simulink subsystem "stewart_strut"  (R2025b)
settings: Solver=VariableStepAuto  StartTime=0.0  StopTime=10.0  RelTol=1e-3
undefined symbols (not defined in the file): DiscIntNeverNeededParam, i, lengthServoConfig, stewart, X, Y, Z
libraries: sm_lib x53, nesl_utility x39
(part 1 of 3)
settings Model: Creator=thomas  LastModifiedBy=David_X
settings SolverCC: AlgebraicLoopSolver=TrustRegion
settings DebuggingCC: UnconnectedInputMsg=warning  UnconnectedOutputMsg=warning  UnconnectedLineMsg=warning
settings ModelReferenceCC: EnableRefExpFcnMdlSchedulingChecks=on
settings RTWCC: GPUComputeCapability=3.5

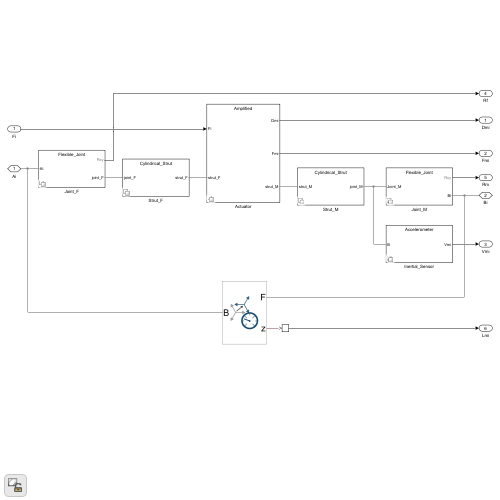
[thumbnail: Simulink's stored preview of the top-level diagram]
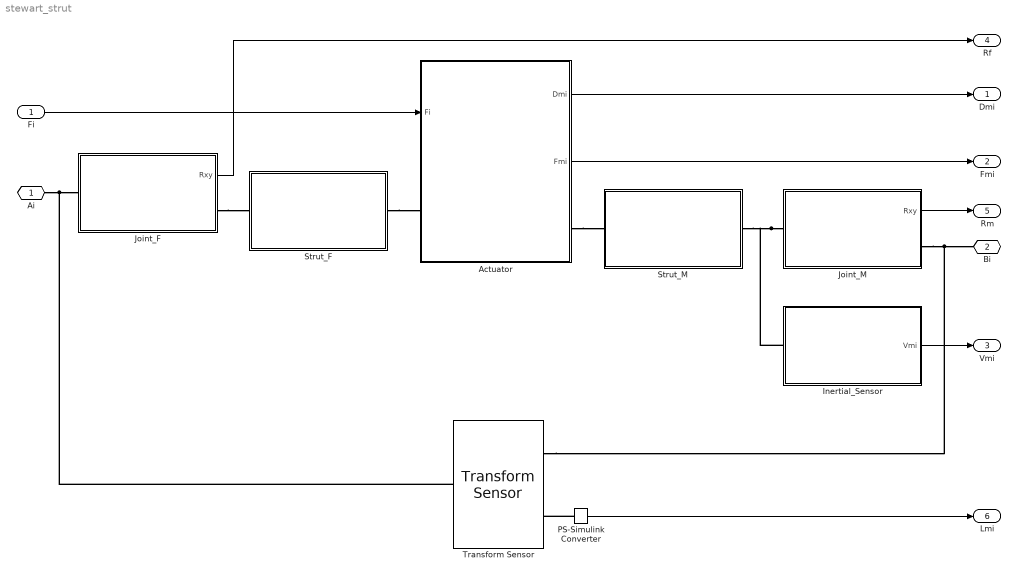
== system stewart_strut ==
  Fi : Inport  Unit=N
  Actuator : Subsystem  Variant=on  VariantControl=Variant1
  Inertial_Sensor : Subsystem  Variant=on  VariantControl=Variant1
  Joint_F : Subsystem  Variant=on  VariantControl=Variant1
  Joint_M : Subsystem  Variant=on  VariantControl=Variant1
  PS-Simulink Converter : nesl_utility/PS-Simulink Converter  PhysicalDomain=network_engine_domain  SubClassName=ps_output  LeftPortType=input  RightPortType=output  PseudoPeriodic=off  Frequencies=[]  VectorFormat=1-D array  Unit=inherit  AffineConversion=off
  Strut_F : Subsystem  Variant=on  VariantControl=Variant1
  Strut_M : Subsystem  Variant=on  VariantControl=Variant1
  Transform Sensor : sm_lib/Frames and Transforms/Transform Sensor  MeasurementFrame=Base  RotationSequence=XYX  SenseAngle=off  SenseAxis=off  SenseQ=off  SenseR=off  SenseRotationSequence=off  SenseOmegaX=off  SenseOmegaY=off  SenseOmegaZ=off  SenseOmega=off  SenseQDot=off  SenseRDot=off  SenseRotationSequenceDot=off  SenseAlphaX=off  SenseAlphaY=off  SenseAlphaZ=off  SenseAlpha=off  SenseQDDot=off  SenseRDDot=off  SenseX=off  SenseY=off  SenseZ=on  SenseXYZ=off  SenseRad=off  SenseAzim=off  SenseDist=off  SenseInc=off  SenseXDot=off  SenseYDot=off  SenseZDot=off  SenseXYZDot=off  SenseRadDot=off  SenseAzimDot=off  SenseDistDot=off  SenseIncDot=off  SenseXDDot=off  SenseYDDot=off  SenseZDDot=off  SenseXYZDDot=off  SenseRadDDot=off  SenseAzimDDot=off  SenseDistDDot=off  SenseIncDDot=off
  Ai : PMIOPort  Side=Left
  Bi : PMIOPort  Port=2  Side=Right
  Dmi : Outport
  Fmi : Outport  Port=2
  Vmi : Outport  Port=3
  Rf : Outport  Port=4
  Rm : Outport  Port=5
  Lmi : Outport  Port=6
  wires:
  Inertial_Sensor/1(Vmi) -> Vmi/1
  Actuator/1(Dmi) -> Dmi/1
  Fi/1 -> Actuator/1(Fi)
  Actuator/2(Fmi) -> Fmi/1
  Joint_M/1(Rxy) -> Rm/1
  Joint_F/1(Rxy) -> Rf/1
  PS-Simulink Converter/1 -> Lmi/1
  connections:
  Transform Sensor/LConn1 -- Ai/RConn1 -- Joint_F/LConn1
  Transform Sensor/RConn1 -- Joint_M/RConn1 -- Bi/RConn1
  Joint_M/LConn1 -- Strut_M/RConn1 -- Inertial_Sensor/LConn1
  Actuator/RConn1 -- Strut_M/LConn1
  Joint_F/RConn1 -- Strut_F/LConn1
  Strut_F/RConn1 -- Actuator/LConn1
  PS-Simulink Converter/LConn1 -- Transform Sensor/RConn2

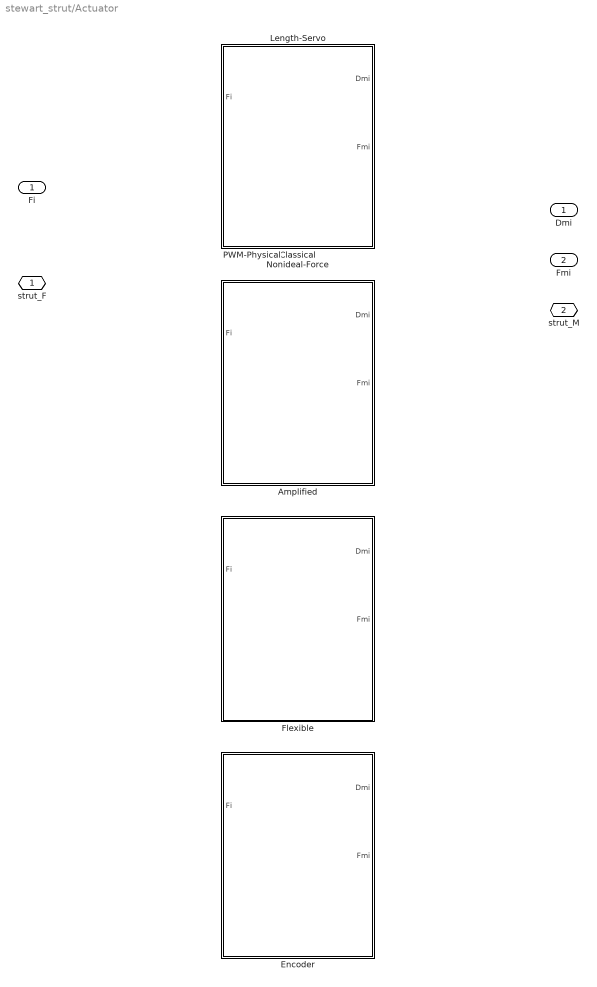
== system stewart_strut/Actuator ==
  Fi : Inport
  Amplified : Subsystem  VariantControl=stewart.actuators.type==2
  Classical : Subsystem  VariantControl=stewart.actuators.type==1
  Encoder : Subsystem  VariantControl=stewart.actuators.type==4
  Flexible : Subsystem  VariantControl=stewart.actuators.type==3
  Length-Servo : Subsystem  VariantControl=stewart.actuators.type==5
  Nonideal-Force : Subsystem  VariantControl=stewart.actuators.type==7
  PWM-Physical : Subsystem  VariantControl=stewart.actuators.type==6
  strut_F : PMIOPort  Side=Left
  strut_M : PMIOPort  Port=2  Side=Right
  Dmi : Outport
  Fmi : Outport  Port=2

== system stewart_strut/Inertial_Sensor ==
  Accelerometer : Subsystem  VariantControl=stewart.sensors.inertial.type == 2
  Geophone : Subsystem  VariantControl=stewart.sensors.inertial.type == 1
  None : Subsystem  VariantControl=stewart.sensors.inertial.type == 3
  B : PMIOPort  Side=Left
  Vmi : Outport

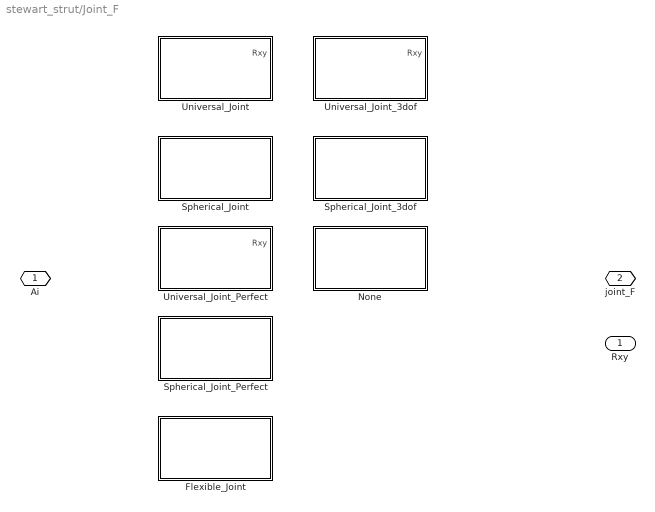
== system stewart_strut/Joint_F ==
  Flexible_Joint : Subsystem  VariantControl=stewart.joints_F.type == 5
  None : Subsystem  VariantControl=stewart.joints_F.type == 10
  Spherical_Joint : Subsystem  VariantControl=stewart.joints_F.type == 2
  Spherical_Joint_3dof : Subsystem  VariantControl=stewart.joints_F.type == 7
  Spherical_Joint_Perfect : Subsystem  VariantControl=stewart.joints_F.type == 4
  Universal_Joint : Subsystem  VariantControl=stewart.joints_F.type == 1
  Universal_Joint_3dof : Subsystem  VariantControl=stewart.joints_F.type == 6
  Universal_Joint_Perfect : Subsystem  VariantControl=stewart.joints_F.type == 3
  Ai : PMIOPort  Side=Left
  joint_F : PMIOPort  Port=2  Side=Right
  Rxy : Outport

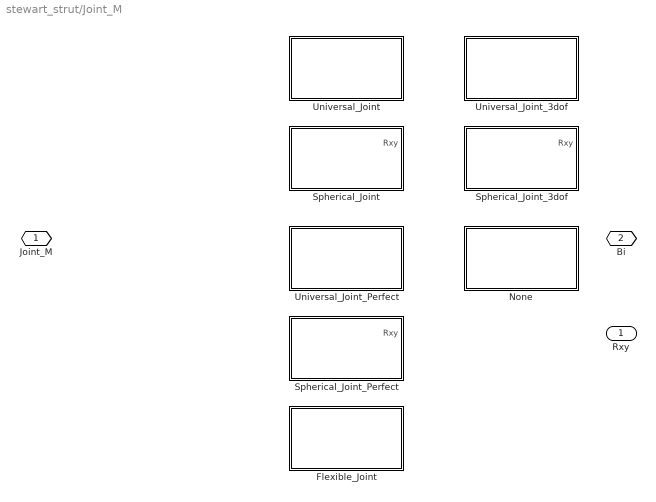
== system stewart_strut/Joint_M ==
  Flexible_Joint : Subsystem  VariantControl=stewart.joints_M.type == 5
  None : Subsystem  VariantControl=stewart.joints_M.type == 10
  Spherical_Joint : Subsystem  VariantControl=stewart.joints_M.type == 2
  Spherical_Joint_3dof : Subsystem  VariantControl=stewart.joints_M.type == 7
  Spherical_Joint_Perfect : Subsystem  VariantControl=stewart.joints_M.type == 4
  Universal_Joint : Subsystem  VariantControl=stewart.joints_M.type == 1
  Universal_Joint_3dof : Subsystem  VariantControl=stewart.joints_M.type == 6
  Universal_Joint_Perfect : Subsystem  VariantControl=stewart.joints_M.type == 3
  Joint_M : PMIOPort  Side=Left
  Bi : PMIOPort  Port=2  Side=Right
  Rxy : Outport

== system stewart_strut/Strut_F ==
  Cylindrical_Strut : Subsystem  VariantControl=stewart.struts_F.type == 1
  None : Subsystem  VariantControl=stewart.struts_F.type == 2
  Null : Subsystem  VariantControl=stewart.struts_F.type == 3
  joint_F : PMIOPort  Side=Left
  strut_F : PMIOPort  Port=2  Side=Right

== system stewart_strut/Strut_M ==
  Cylindrical_Strut : Subsystem  VariantControl=stewart.struts_F.type == 1
  None : Subsystem  VariantControl=stewart.struts_F.type == 2
  Null : Subsystem  VariantControl=stewart.struts_F.type == 3
  strut_M : PMIOPort  Side=Left
  joint_M : PMIOPort  Port=2  Side=Right

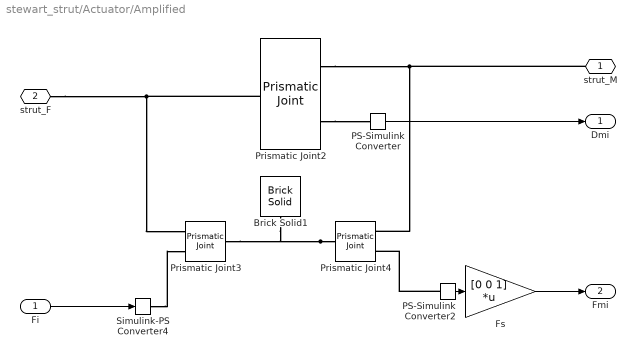
== system stewart_strut/Actuator/Amplified ==
  Fi : Inport
  Brick Solid1 : sm_lib/Body Elements/Brick Solid  BrickDimensions=[1 1 1.5]  BrickDimensionsUnits=cm  ExportEntireGeometry=off  InertiaType=CalculateFromGeometry  BasedOnType=Mass  Density=1000  DensityUnits=kg/m^3  Mass=0.001  MassUnits=kg  CenterOfMass=[0 0 0]  CenterOfMassUnits=m  MomentsOfInertia=[1 1 1]  MomentsOfInertiaUnits=kg*m^2  ProductsOfInertia=[0 0 0]  ProductsOfInertiaUnits=kg*m^2  GraphicType=FromGeometry  MarkerShape=Sphere  MarkerSize=10  GraphicVisPropType=SimpleVisualProperties  GraphicDiffuseColor=[0.5 0.5 0.5]  GraphicOpacity=1.0  GraphicSpecularColor=[0.5 0.5 0.5 1.0]  GraphicAmbientColor=[0.15 0.15 0.15 1.0]  GraphicEmissiveColor=[0.0 0.0 0.0 1.0]  GraphicShininess=75  DoExposeReferenceFrame=on  SerializedFrames=<Frames/>
  Fs : Gain  Gain=[0 0 1]  Multiplication=Matrix(K*u)
  PS-Simulink Converter : nesl_utility/PS-Simulink Converter  PhysicalDomain=network_engine_domain  SubClassName=ps_output  LeftPortType=input  RightPortType=output  PseudoPeriodic=off  Frequencies=[]  VectorFormat=1-D array  Unit=m  AffineConversion=off
  PS-Simulink Converter2 : nesl_utility/PS-Simulink Converter  PhysicalDomain=network_engine_domain  SubClassName=ps_output  LeftPortType=input  RightPortType=output  PseudoPeriodic=off  Frequencies=[]  VectorFormat=1-D array  Unit=N  AffineConversion=off
  Prismatic Joint2 : sm_lib/Joints/Prismatic Joint  JointMode=Normal  CompositeWrenchDir=FollowerOnBase  CompositeWrenchFrame=BaseFrame  SenseConstraintForce=off  SenseConstraintTorque=off  SenseTotalForce=off  SenseTotalTorque=off  PositionTargetSpecify=off  PositionTargetPriority=High  PositionTargetValue=0  PositionTargetValueUnits=m  VelocityTargetSpecify=off  VelocityTargetPriority=High  VelocityTargetValue=0  VelocityTargetValueUnits=m/s  EquilibriumPosition=stewart.actuators.Leq(i)  EquilibriumPositionUnits=m  SpringStiffness=stewart.actuators.K1(i)  SpringStiffnessUnits=N/m  DampingCoefficient=stewart.actuators.C1(i)  DampingCoefficientUnits=N/(m/s)  LowerLimitSpecify=off  LowerLimitBound=-1  LowerLimitBoundUnits=m  LowerLimitStiffness=1e6  LowerLimitStiffnessUnits=N/m  LowerLimitDamping=1e3  LowerLimitDampingUnits=N/(m/s)  LowerLimitTransitionRegionWidth=1e-4  LowerLimitTransitionRegionWidthUnits=m  UpperLimitSpecify=off  UpperLimitBound=1  UpperLimitBoundUnits=m  UpperLimitStiffness=1e6  UpperLimitStiffnessUnits=N/m  UpperLimitDamping=1e3  UpperLimitDampingUnits=N/(m/s)  UpperLimitTransitionRegionWidth=1e-4  UpperLimitTransitionRegionWidthUnits=m  TorqueActuationMode=NoTorque  MotionActuationMode=ComputedMotion  SensePosition=on  SenseVelocity=off  SenseAcceleration=off  SenseTorqueForce=off  SenseLowerLimitTorqueForce=off  SenseUpperLimitTorqueForce=off
  Prismatic Joint3 : sm_lib/Joints/Prismatic Joint  JointMode=Normal  CompositeWrenchDir=FollowerOnBase  CompositeWrenchFrame=BaseFrame  SenseConstraintForce=off  SenseConstraintTorque=off  SenseTotalForce=off  SenseTotalTorque=off  PositionTargetSpecify=off  PositionTargetPriority=Low  PositionTargetValue=0  PositionTargetValueUnits=m  VelocityTargetSpecify=off  VelocityTargetPriority=High  VelocityTargetValue=0  VelocityTargetValueUnits=m/s  EquilibriumPosition=0  EquilibriumPositionUnits=m  SpringStiffness=stewart.actuators.Ka(i)  SpringStiffnessUnits=N/m  DampingCoefficient=0  DampingCoefficientUnits=N/(m/s)  LowerLimitSpecify=off  LowerLimitBound=-1  LowerLimitBoundUnits=m  LowerLimitStiffness=1e6  LowerLimitStiffnessUnits=N/m  LowerLimitDamping=1e3  LowerLimitDampingUnits=N/(m/s)  LowerLimitTransitionRegionWidth=1e-4  LowerLimitTransitionRegionWidthUnits=m  UpperLimitSpecify=off  UpperLimitBound=1  UpperLimitBoundUnits=m  UpperLimitStiffness=1e6  UpperLimitStiffnessUnits=N/m  UpperLimitDamping=1e3  UpperLimitDampingUnits=N/(m/s)  UpperLimitTransitionRegionWidth=1e-4  UpperLimitTransitionRegionWidthUnits=m  TorqueActuationMode=InputTorque  MotionActuationMode=ComputedMotion  SensePosition=off  SenseVelocity=off  SenseAcceleration=off  SenseTorqueForce=off  SenseLowerLimitTorqueForce=off  SenseUpperLimitTorqueForce=off
  Prismatic Joint4 : sm_lib/Joints/Prismatic Joint  JointMode=Normal  CompositeWrenchDir=FollowerOnBase  CompositeWrenchFrame=BaseFrame  SenseConstraintForce=off  SenseConstraintTorque=off  SenseTotalForce=on  SenseTotalTorque=off  PositionTargetSpecify=off  PositionTargetPriority=Low  PositionTargetValue=0  PositionTargetValueUnits=m  VelocityTargetSpecify=off  VelocityTargetPriority=High  VelocityTargetValue=0  VelocityTargetValueUnits=m/s  EquilibriumPosition=0  EquilibriumPositionUnits=m  SpringStiffness=stewart.actuators.Ke(i)  SpringStiffnessUnits=N/m  DampingCoefficient=0  DampingCoefficientUnits=N/(m/s)  LowerLimitSpecify=off  LowerLimitBound=-1  LowerLimitBoundUnits=m  LowerLimitStiffness=1e6  LowerLimitStiffnessUnits=N/m  LowerLimitDamping=1e3  LowerLimitDampingUnits=N/(m/s)  LowerLimitTransitionRegionWidth=1e-4  LowerLimitTransitionRegionWidthUnits=m  UpperLimitSpecify=off  UpperLimitBound=1  UpperLimitBoundUnits=m  UpperLimitStiffness=1e6  UpperLimitStiffnessUnits=N/m  UpperLimitDamping=1e3  UpperLimitDampingUnits=N/(m/s)  UpperLimitTransitionRegionWidth=1e-4  UpperLimitTransitionRegionWidthUnits=m  TorqueActuationMode=NoTorque  MotionActuationMode=ComputedMotion  SensePosition=off  SenseVelocity=off  SenseAcceleration=off  SenseTorqueForce=off  SenseLowerLimitTorqueForce=off  SenseUpperLimitTorqueForce=off
  Simulink-PS Converter4 : nesl_utility/Simulink-PS Converter  PhysicalDomain=network_engine_domain  SubClassName=ps_input  LeftPortType=input  RightPortType=output  PseudoPeriodic=off  Frequencies=[]  NoiseDistribution=none  NoiseParameters=[]  Unit=N  AffineConversion=off  FilteringAndDerivatives=provide  SimscapeFilterOrder=1  InputFilterTimeConstant=0.001  UdotUserProvided=0
  strut_M : PMIOPort  Side=Right
  strut_F : PMIOPort  Port=2  Side=Left
  Dmi : Outport
  Fmi : Outport  Port=2
  wires:
  PS-Simulink Converter/1 -> Dmi/1
  PS-Simulink Converter2/1 -> Fs/1
  Fi/1 -> Simulink-PS Converter4/1
  Fs/1 -> Fmi/1
  connections:
  strut_M/RConn1 -- Prismatic Joint2/RConn1 -- Prismatic Joint4/RConn1
  Prismatic Joint2/LConn1 -- Prismatic Joint3/LConn1 -- strut_F/RConn1
  PS-Simulink Converter2/LConn1 -- Prismatic Joint4/RConn2
  Simulink-PS Converter4/RConn1 -- Prismatic Joint3/LConn2
  Prismatic Joint2/RConn2 -- PS-Simulink Converter/LConn1
  Prismatic Joint4/LConn1 -- Prismatic Joint3/RConn1 -- Brick Solid1/RConn1

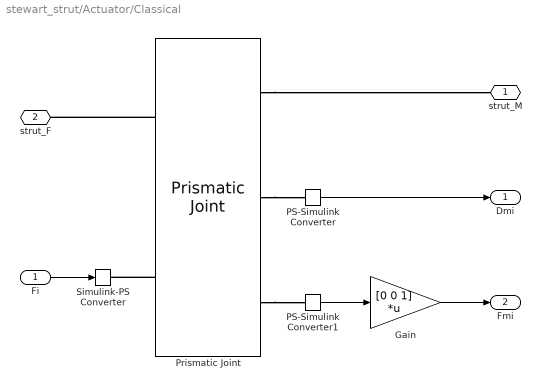
== system stewart_strut/Actuator/Classical ==
  Fi : Inport
  Gain : Gain  Gain=[0 0 1]  Multiplication=Matrix(K*u)
  PS-Simulink Converter : nesl_utility/PS-Simulink Converter  PhysicalDomain=network_engine_domain  SubClassName=ps_output  LeftPortType=input  RightPortType=output  PseudoPeriodic=off  Frequencies=[]  VectorFormat=1-D array  Unit=m  AffineConversion=off
  PS-Simulink Converter1 : nesl_utility/PS-Simulink Converter  PhysicalDomain=network_engine_domain  SubClassName=ps_output  LeftPortType=input  RightPortType=output  PseudoPeriodic=off  Frequencies=[]  VectorFormat=1-D array  Unit=N  AffineConversion=on
  Prismatic Joint : sm_lib/Joints/Prismatic Joint  JointMode=Normal  CompositeWrenchDir=BaseOnFollower  CompositeWrenchFrame=BaseFrame  SenseConstraintForce=off  SenseConstraintTorque=off  SenseTotalForce=on  SenseTotalTorque=off  PositionTargetSpecify=on  PositionTargetPriority=High  PositionTargetValue=stewart.actuators.Leq(i)  PositionTargetValueUnits=m  VelocityTargetSpecify=off  VelocityTargetPriority=High  VelocityTargetValue=0  VelocityTargetValueUnits=m/s  EquilibriumPosition=stewart.actuators.Leq(i)  EquilibriumPositionUnits=m  SpringStiffness=stewart.actuators.K(i)  SpringStiffnessUnits=N/m  DampingCoefficient=stewart.actuators.C(i)  DampingCoefficientUnits=N/(m/s)  LowerLimitSpecify=off  LowerLimitBound=-1  LowerLimitBoundUnits=m  LowerLimitStiffness=1e6  LowerLimitStiffnessUnits=N/m  LowerLimitDamping=1e3  LowerLimitDampingUnits=N/(m/s)  LowerLimitTransitionRegionWidth=1e-4  LowerLimitTransitionRegionWidthUnits=m  UpperLimitSpecify=off  UpperLimitBound=1  UpperLimitBoundUnits=m  UpperLimitStiffness=1e6  UpperLimitStiffnessUnits=N/m  UpperLimitDamping=1e3  UpperLimitDampingUnits=N/(m/s)  UpperLimitTransitionRegionWidth=1e-4  UpperLimitTransitionRegionWidthUnits=m  TorqueActuationMode=InputTorque  MotionActuationMode=ComputedMotion  SensePosition=on  SenseVelocity=off  SenseAcceleration=off  SenseTorqueForce=off  SenseLowerLimitTorqueForce=off  SenseUpperLimitTorqueForce=off
  Simulink-PS Converter : nesl_utility/Simulink-PS Converter  PhysicalDomain=network_engine_domain  SubClassName=ps_input  LeftPortType=input  RightPortType=output  PseudoPeriodic=off  Frequencies=[]  NoiseDistribution=none  NoiseParameters=[]  Unit=N  AffineConversion=off  FilteringAndDerivatives=provide  SimscapeFilterOrder=1  InputFilterTimeConstant=0.001  UdotUserProvided=0
  strut_M : PMIOPort  Side=Right
  strut_F : PMIOPort  Port=2  Side=Left
  Dmi : Outport
  Fmi : Outport  Port=2
  wires:
  Gain/1 -> Fmi/1
  Fi/1 -> Simulink-PS Converter/1
  PS-Simulink Converter1/1 -> Gain/1
  PS-Simulink Converter/1 -> Dmi/1
  connections:
  Prismatic Joint/RConn3 -- PS-Simulink Converter1/LConn1
  Prismatic Joint/RConn2 -- PS-Simulink Converter/LConn1
  Prismatic Joint/RConn1 -- strut_M/RConn1
  Prismatic Joint/LConn2 -- Simulink-PS Converter/RConn1
  Prismatic Joint/LConn1 -- strut_F/RConn1

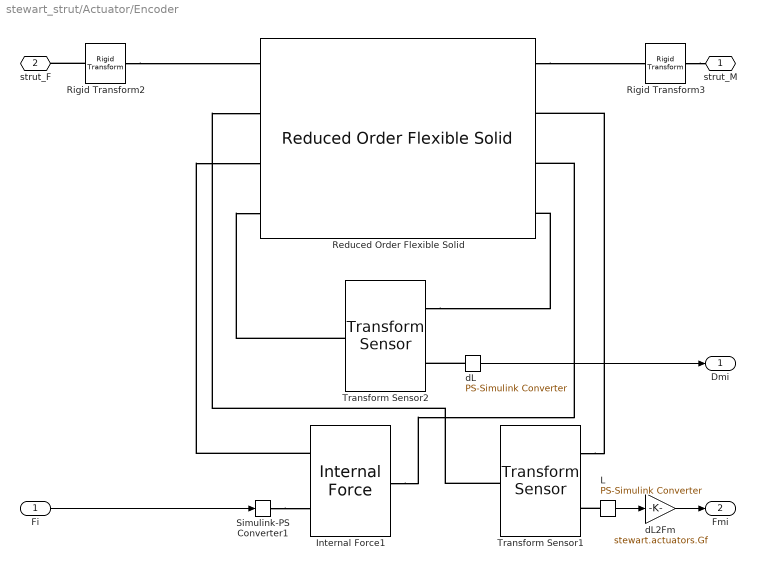
== system stewart_strut/Actuator/Encoder ==
  Fi : Inport
  Internal Force1 : sm_lib/Forces and Torques/Internal Force
  L : nesl_utility/PS-Simulink Converter  PhysicalDomain=network_engine_domain  SubClassName=ps_output  LeftPortType=input  RightPortType=output  PseudoPeriodic=off  Frequencies=[]  VectorFormat=1-D array  Unit=m  AffineConversion=off
  Reduced Order Flexible Solid : sm_lib/Body Elements/Flexible Bodies/Reduced Order Flexible Solid  UnitSystemType=SI  LengthUnit=m  MassUnit=kg  TimeUnit=s  NumberOfInterfaceFrames=8  InterfaceFrameOrigins=stewart.actuators.n_xyz  InterfaceFrameOrientations=repmat([1 0 0 0],8,1)  StiffnessMatrix=stewart.actuators.Km  MassMatrix=stewart.actuators.Mm  DampingType=UniformModal  ProportionalDampingAlpha=1e-6  ProportionalDampingBeta=3e-6  UniformModalDampingRatio=stewart.actuators.xi  DampingMatrix=[]  ReferenceConditionsType=LinearizedMeanAxes  DoExposeReferenceFrame=off  ReductionType=None  NumRetainedModes=1  GraphicType=PartitionedGeometry  GeomFileName=./mat/strut_encoder.step  GeomUnitType=FromFile  VisRecursionLimit=3  GraphicVertexCoordinates=[]  GraphicFacetVertexIndices=[]  GraphicReconstructionMatrix=[]  GraphicVisPropType=SimpleVisualProperties  GraphicDiffuseColor=[0.2 0.4 1.0]  GraphicOpacity=1.0  GraphicSpecularColor=[0.5 0.5 0.5 1.0]  GraphicAmbientColor=[0.15 0.15 0.15 1.0]  GraphicEmissiveColor=[0.0 0.0 0.0 1.0]  GraphicShininess=75
  Rigid Transform2 : sm_lib/Frames and Transforms/Rigid Transform  RotationMethod=None  FollAlignAxisA=+X  BaseAlignAxisA=+Y  FollAlignAxisB=+Y  BaseAlignAxisB=+Z  RotationStandardAxis=+Z  RotationAngle=0.0  RotationAngleUnits=deg  RotationArbitraryAxis=[0 0 1]  RotationSequenceAxes=FollowerAxes  RotationSequence=XYX  RotationSequenceAngles=[0 0 0]  RotationSequenceAnglesUnits=deg  RotationMatrix=[1 0 0; 0 1 0; 0 0 1]  Quaternion=[1 0 0 0]  TranslationMethod=StandardAxis  TranslationCartesianOffset=[0 0 0]  TranslationCartesianOffsetUnits=m  TranslationStandardAxis=+Z  TranslationStandardOffset=stewart.actuators.ax_off  TranslationStandardOffsetUnits=m  TranslationROffset=0  TranslationROffsetUnits=m  TranslationThetaOffset=0  TranslationThetaOffsetUnits=deg  TranslationZOffset=0  TranslationZOffsetUnits=m
  Rigid Transform3 : sm_lib/Frames and Transforms/Rigid Transform  RotationMethod=None  FollAlignAxisA=+X  BaseAlignAxisA=+Y  FollAlignAxisB=+Y  BaseAlignAxisB=+Z  RotationStandardAxis=+Z  RotationAngle=0.0  RotationAngleUnits=deg  RotationArbitraryAxis=[0 0 1]  RotationSequenceAxes=FollowerAxes  RotationSequence=XYX  RotationSequenceAngles=[0 0 0]  RotationSequenceAnglesUnits=deg  RotationMatrix=[1 0 0; 0 1 0; 0 0 1]  Quaternion=[1 0 0 0]  TranslationMethod=StandardAxis  TranslationCartesianOffset=[0 0 0]  TranslationCartesianOffsetUnits=m  TranslationStandardAxis=+Z  TranslationStandardOffset=stewart.actuators.ax_off  TranslationStandardOffsetUnits=m  TranslationROffset=0  TranslationROffsetUnits=m  TranslationThetaOffset=0  TranslationThetaOffsetUnits=deg  TranslationZOffset=0  TranslationZOffsetUnits=m
  Simulink-PS Converter1 : nesl_utility/Simulink-PS Converter  PhysicalDomain=network_engine_domain  SubClassName=ps_input  LeftPortType=input  RightPortType=output  PseudoPeriodic=off  Frequencies=[]  NoiseDistribution=none  NoiseParameters=[]  Unit=N  AffineConversion=off  FilteringAndDerivatives=provide  SimscapeFilterOrder=1  InputFilterTimeConstant=0.001  UdotUserProvided=0
  Transform Sensor1 : sm_lib/Frames and Transforms/Transform Sensor  MeasurementFrame=Base  RotationSequence=XYX  SenseAngle=off  SenseAxis=off  SenseQ=off  SenseR=off  SenseRotationSequence=off  SenseOmegaX=off  SenseOmegaY=off  SenseOmegaZ=off  SenseOmega=off  SenseQDot=off  SenseRDot=off  SenseRotationSequenceDot=off  SenseAlphaX=off  SenseAlphaY=off  SenseAlphaZ=off  SenseAlpha=off  SenseQDDot=off  SenseRDDot=off  SenseX=on  SenseY=off  SenseZ=off  SenseXYZ=off  SenseRad=off  SenseAzim=off  SenseDist=off  SenseInc=off  SenseXDot=off  SenseYDot=off  SenseZDot=off  SenseXYZDot=off  SenseRadDot=off  SenseAzimDot=off  SenseDistDot=off  SenseIncDot=off  SenseXDDot=off  SenseYDDot=off  SenseZDDot=off  SenseXYZDDot=off  SenseRadDDot=off  SenseAzimDDot=off  SenseDistDDot=off  SenseIncDDot=off
  Transform Sensor2 : sm_lib/Frames and Transforms/Transform Sensor  MeasurementFrame=Base  RotationSequence=XYX  SenseAngle=off  SenseAxis=off  SenseQ=off  SenseR=off  SenseRotationSequence=off  SenseOmegaX=off  SenseOmegaY=off  SenseOmegaZ=off  SenseOmega=off  SenseQDot=off  SenseRDot=off  SenseRotationSequenceDot=off  SenseAlphaX=off  SenseAlphaY=off  SenseAlphaZ=off  SenseAlpha=off  SenseQDDot=off  SenseRDDot=off  SenseX=off  SenseY=off  SenseZ=on  SenseXYZ=off  SenseRad=off  SenseAzim=off  SenseDist=off  SenseInc=off  SenseXDot=off  SenseYDot=off  SenseZDot=off  SenseXYZDot=off  SenseRadDot=off  SenseAzimDot=off  SenseDistDot=off  SenseIncDot=off  SenseXDDot=off  SenseYDDot=off  SenseZDDot=off  SenseXYZDDot=off  SenseRadDDot=off  SenseAzimDDot=off  SenseDistDDot=off  SenseIncDDot=off
  dL : nesl_utility/PS-Simulink Converter  PhysicalDomain=network_engine_domain  SubClassName=ps_output  LeftPortType=input  RightPortType=output  PseudoPeriodic=off  Frequencies=[]  VectorFormat=1-D array  Unit=m  AffineConversion=off
  dL2Fm : Gain  Gain=stewart.actuators.Gf
  strut_M : PMIOPort  Side=Right
  strut_F : PMIOPort  Port=2  Side=Left
  Dmi : Outport
  Fmi : Outport  Port=2
  wires:
  dL/1 -> Dmi/1
  dL2Fm/1 -> Fmi/1
  Fi/1 -> Simulink-PS Converter1/1
  L/1 -> dL2Fm/1
  connections:
  Transform Sensor2/LConn1 -- Reduced Order Flexible Solid/RConn4
  Reduced Order Flexible Solid/LConn1 -- Rigid Transform3/LConn1
  Rigid Transform2/RConn1 -- Reduced Order Flexible Solid/RConn1
  dL/LConn1 -- Transform Sensor2/RConn2
  Transform Sensor2/RConn1 -- Reduced Order Flexible Solid/LConn4
  Transform Sensor1/RConn1 -- Reduced Order Flexible Solid/LConn2
  Transform Sensor1/LConn1 -- Reduced Order Flexible Solid/RConn2
  Internal Force1/RConn1 -- Reduced Order Flexible Solid/LConn3
  Internal Force1/LConn1 -- Reduced Order Flexible Solid/RConn3
  Rigid Transform2/LConn1 -- strut_F/RConn1
  Rigid Transform3/RConn1 -- strut_M/RConn1
  L/LConn1 -- Transform Sensor1/RConn2
  Simulink-PS Converter1/RConn1 -- Internal Force1/LConn2

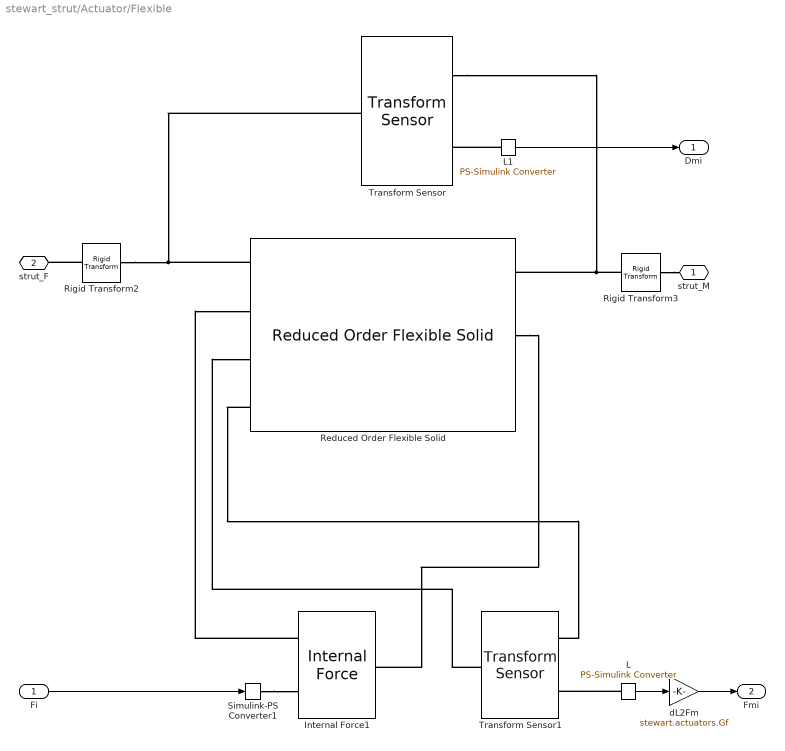
== system stewart_strut/Actuator/Flexible ==
  Fi : Inport
  Internal Force1 : sm_lib/Forces and Torques/Internal Force
  L : nesl_utility/PS-Simulink Converter  PhysicalDomain=network_engine_domain  SubClassName=ps_output  LeftPortType=input  RightPortType=output  PseudoPeriodic=off  Frequencies=[]  VectorFormat=1-D array  Unit=m  AffineConversion=off
  L1 : nesl_utility/PS-Simulink Converter  PhysicalDomain=network_engine_domain  SubClassName=ps_output  LeftPortType=input  RightPortType=output  PseudoPeriodic=off  Frequencies=[]  VectorFormat=1-D array  Unit=inherit  AffineConversion=off
  Reduced Order Flexible Solid : sm_lib/Body Elements/Flexible Bodies/Reduced Order Flexible Solid  UnitSystemType=SI  LengthUnit=m  MassUnit=kg  TimeUnit=s  NumberOfInterfaceFrames=7  InterfaceFrameOrigins=stewart.actuators.n_xyz  InterfaceFrameOrientations=repmat([1 0 0 0],7,1)  StiffnessMatrix=stewart.actuators.Km  MassMatrix=stewart.actuators.Mm  DampingType=UniformModal  ProportionalDampingAlpha=1e-6  ProportionalDampingBeta=3e-6  UniformModalDampingRatio=stewart.actuators.xi  DampingMatrix=[]  ReferenceConditionsType=LinearizedMeanAxes  DoExposeReferenceFrame=off  ReductionType=None  NumRetainedModes=1  GraphicType=PartitionedGeometry  GeomFileName=./mat/APA300ML.STEP  GeomUnitType=FromFile  VisRecursionLimit=3  GraphicVertexCoordinates=[]  GraphicFacetVertexIndices=[]  GraphicReconstructionMatrix=[]  GraphicVisPropType=SimpleVisualProperties  GraphicDiffuseColor=[0.2 0.4 1.0]  GraphicOpacity=1.0  GraphicSpecularColor=[0.5 0.5 0.5 1.0]  GraphicAmbientColor=[0.15 0.15 0.15 1.0]  GraphicEmissiveColor=[0.0 0.0 0.0 1.0]  GraphicShininess=75
  Rigid Transform2 : sm_lib/Frames and Transforms/Rigid Transform  RotationMethod=None  FollAlignAxisA=+X  BaseAlignAxisA=+Y  FollAlignAxisB=+Y  BaseAlignAxisB=+Z  RotationStandardAxis=+Z  RotationAngle=0.0  RotationAngleUnits=deg  RotationArbitraryAxis=[0 0 1]  RotationSequenceAxes=FollowerAxes  RotationSequence=XYX  RotationSequenceAngles=[0 0 0]  RotationSequenceAnglesUnits=deg  RotationMatrix=[1 0 0; 0 1 0; 0 0 1]  Quaternion=[1 0 0 0]  TranslationMethod=StandardAxis  TranslationCartesianOffset=[0 0 0]  TranslationCartesianOffsetUnits=m  TranslationStandardAxis=+Z  TranslationStandardOffset=stewart.actuators.ax_off  TranslationStandardOffsetUnits=m  TranslationROffset=0  TranslationROffsetUnits=m  TranslationThetaOffset=0  TranslationThetaOffsetUnits=deg  TranslationZOffset=0  TranslationZOffsetUnits=m
  Rigid Transform3 : sm_lib/Frames and Transforms/Rigid Transform  RotationMethod=None  FollAlignAxisA=+X  BaseAlignAxisA=+Y  FollAlignAxisB=+Y  BaseAlignAxisB=+Z  RotationStandardAxis=+Z  RotationAngle=0.0  RotationAngleUnits=deg  RotationArbitraryAxis=[0 0 1]  RotationSequenceAxes=FollowerAxes  RotationSequence=XYX  RotationSequenceAngles=[0 0 0]  RotationSequenceAnglesUnits=deg  RotationMatrix=[1 0 0; 0 1 0; 0 0 1]  Quaternion=[1 0 0 0]  TranslationMethod=StandardAxis  TranslationCartesianOffset=[0 0 0]  TranslationCartesianOffsetUnits=m  TranslationStandardAxis=+Z  TranslationStandardOffset=stewart.actuators.ax_off  TranslationStandardOffsetUnits=m  TranslationROffset=0  TranslationROffsetUnits=m  TranslationThetaOffset=0  TranslationThetaOffsetUnits=deg  TranslationZOffset=0  TranslationZOffsetUnits=m
  Simulink-PS Converter1 : nesl_utility/Simulink-PS Converter  PhysicalDomain=network_engine_domain  SubClassName=ps_input  LeftPortType=input  RightPortType=output  PseudoPeriodic=off  Frequencies=[]  NoiseDistribution=none  NoiseParameters=[]  Unit=N  AffineConversion=off  FilteringAndDerivatives=provide  SimscapeFilterOrder=1  InputFilterTimeConstant=0.001  UdotUserProvided=0
  Transform Sensor : sm_lib/Frames and Transforms/Transform Sensor  MeasurementFrame=Base  RotationSequence=XYX  SenseAngle=off  SenseAxis=off  SenseQ=off  SenseR=off  SenseRotationSequence=off  SenseOmegaX=off  SenseOmegaY=off  SenseOmegaZ=off  SenseOmega=off  SenseQDot=off  SenseRDot=off  SenseRotationSequenceDot=off  SenseAlphaX=off  SenseAlphaY=off  SenseAlphaZ=off  SenseAlpha=off  SenseQDDot=off  SenseRDDot=off  SenseX=off  SenseY=off  SenseZ=on  SenseXYZ=off  SenseRad=off  SenseAzim=off  SenseDist=off  SenseInc=off  SenseXDot=off  SenseYDot=off  SenseZDot=off  SenseXYZDot=off  SenseRadDot=off  SenseAzimDot=off  SenseDistDot=off  SenseIncDot=off  SenseXDDot=off  SenseYDDot=off  SenseZDDot=off  SenseXYZDDot=off  SenseRadDDot=off  SenseAzimDDot=off  SenseDistDDot=off  SenseIncDDot=off
  Transform Sensor1 : sm_lib/Frames and Transforms/Transform Sensor  MeasurementFrame=Base  RotationSequence=XYX  SenseAngle=off  SenseAxis=off  SenseQ=off  SenseR=off  SenseRotationSequence=off  SenseOmegaX=off  SenseOmegaY=off  SenseOmegaZ=off  SenseOmega=off  SenseQDot=off  SenseRDot=off  SenseRotationSequenceDot=off  SenseAlphaX=off  SenseAlphaY=off  SenseAlphaZ=off  SenseAlpha=off  SenseQDDot=off  SenseRDDot=off  SenseX=on  SenseY=off  SenseZ=off  SenseXYZ=off  SenseRad=off  SenseAzim=off  SenseDist=off  SenseInc=off  SenseXDot=off  SenseYDot=off  SenseZDot=off  SenseXYZDot=off  SenseRadDot=off  SenseAzimDot=off  SenseDistDot=off  SenseIncDot=off  SenseXDDot=off  SenseYDDot=off  SenseZDDot=off  SenseXYZDDot=off  SenseRadDDot=off  SenseAzimDDot=off  SenseDistDDot=off  SenseIncDDot=off
  dL2Fm : Gain  Gain=stewart.actuators.Gf
  strut_M : PMIOPort  Side=Right
  strut_F : PMIOPort  Port=2  Side=Left
  Dmi : Outport
  Fmi : Outport  Port=2
  wires:
  L/1 -> dL2Fm/1
  Fi/1 -> Simulink-PS Converter1/1
  L1/1 -> Dmi/1
  dL2Fm/1 -> Fmi/1
  connections:
  Reduced Order Flexible Solid/LConn4 -- Transform Sensor1/RConn1
  Internal Force1/LConn1 -- Reduced Order Flexible Solid/LConn2
  Reduced Order Flexible Solid/RConn2 -- Internal Force1/RConn1
  Simulink-PS Converter1/RConn1 -- Internal Force1/LConn2
  Transform Sensor1/LConn1 -- Reduced Order Flexible Solid/LConn3
  Transform Sensor/LConn1 -- Rigid Transform2/RConn1 -- Reduced Order Flexible Solid/LConn1
  L/LConn1 -- Transform Sensor1/RConn2
  Transform Sensor/RConn1 -- Reduced Order Flexible Solid/RConn1 -- Rigid Transform3/LConn1
  Rigid Transform3/RConn1 -- strut_M/RConn1
  L1/LConn1 -- Transform Sensor/RConn2
  Rigid Transform2/LConn1 -- strut_F/RConn1

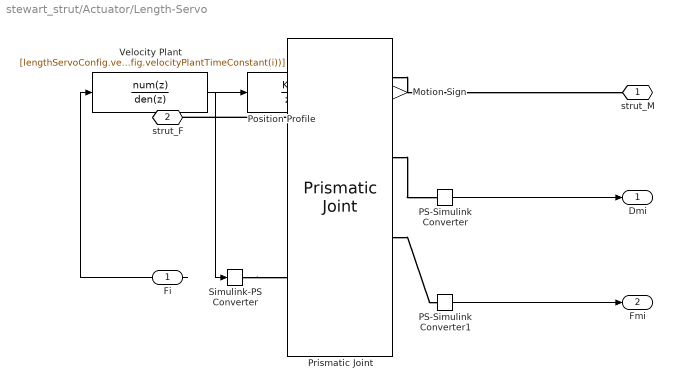
== system stewart_strut/Actuator/Length-Servo ==
  Fi : Inport
  Motion Sign : Gain
  PS-Simulink Converter : nesl_utility/PS-Simulink Converter  PhysicalDomain=network_engine_domain  SubClassName=ps_output  LeftPortType=input  RightPortType=output  PseudoPeriodic=off  Frequencies=[]  VectorFormat=1-D array  Unit=m  AffineConversion=off
  PS-Simulink Converter1 : nesl_utility/PS-Simulink Converter  PhysicalDomain=network_engine_domain  SubClassName=ps_output  LeftPortType=input  RightPortType=output  PseudoPeriodic=off  Frequencies=[]  VectorFormat=1-D array  Unit=m/s  AffineConversion=on
  Position Profile : DiscreteIntegrator  gainval=1  SampleTime=-1  ICPrevOutput=DiscIntNeverNeededParam  ICPrevScaledInput=DiscIntNeverNeededParam
  Prismatic Joint : sm_lib/Joints/Prismatic Joint  JointMode=Normal  CompositeWrenchDir=BaseOnFollower  CompositeWrenchFrame=BaseFrame  SenseConstraintForce=off  SenseConstraintTorque=off  SenseTotalForce=on  SenseTotalTorque=off  PositionTargetSpecify=on  PositionTargetPriority=High  PositionTargetValue=stewart.actuators.Leq(i)  PositionTargetValueUnits=m  VelocityTargetSpecify=off  VelocityTargetPriority=High  VelocityTargetValue=0  VelocityTargetValueUnits=m/s  EquilibriumPosition=stewart.actuators.Leq(i)  EquilibriumPositionUnits=m  SpringStiffness=stewart.actuators.K(i)  SpringStiffnessUnits=N/m  DampingCoefficient=stewart.actuators.C(i)  DampingCoefficientUnits=N/(m/s)  LowerLimitSpecify=off  LowerLimitBound=-1  LowerLimitBoundUnits=m  LowerLimitStiffness=1e6  LowerLimitStiffnessUnits=N/m  LowerLimitDamping=1e3  LowerLimitDampingUnits=N/(m/s)  LowerLimitTransitionRegionWidth=1e-4  LowerLimitTransitionRegionWidthUnits=m  UpperLimitSpecify=off  UpperLimitBound=1  UpperLimitBoundUnits=m  UpperLimitStiffness=1e6  UpperLimitStiffnessUnits=N/m  UpperLimitDamping=1e3  UpperLimitDampingUnits=N/(m/s)  UpperLimitTransitionRegionWidth=1e-4  UpperLimitTransitionRegionWidthUnits=m  TorqueActuationMode=ComputedTorque  MotionActuationMode=InputMotion  SensePosition=on  SenseVelocity=on  SenseAcceleration=off  SenseTorqueForce=off  SenseLowerLimitTorqueForce=off  SenseUpperLimitTorqueForce=off
  Simulink-PS Converter : nesl_utility/Simulink-PS Converter  PhysicalDomain=network_engine_domain  SubClassName=ps_input  LeftPortType=input  RightPortType=output  PseudoPeriodic=off  Frequencies=[]  NoiseDistribution=none  NoiseParameters=[]  Unit=m  AffineConversion=off  FilteringAndDerivatives=filter  SimscapeFilterOrder=2  InputFilterTimeConstant=lengthServoConfig.sampleTime  UdotUserProvided=0
  Velocity Plant : DiscreteTransferFcn  Numerator=[lengthServoConfig.velocityPlantGain(i)*(1-exp(-lengthServoConfig.sampleTime/lengthServoConfig.velocityPlantTimeConstant(i)))]  Denominator=[1 -exp(-lengthServoConfig.sampleTime/lengthServoConfig.velocityPlantTimeConstant(i))]  SampleTime=lengthServoConfig.sampleTime
  strut_M : PMIOPort  Side=Right
  strut_F : PMIOPort  Port=2  Side=Left
  Dmi : Outport
  Fmi : Outport  Port=2
  wires:
  PS-Simulink Converter/1 -> Dmi/1
  Fi/1 -> Velocity Plant/1
  Velocity Plant/1 -> Position Profile/1
  Position Profile/1 -> Motion Sign/1
  Motion Sign/1 -> Simulink-PS Converter/1
  PS-Simulink Converter1/1 -> Fmi/1
  connections:
  Prismatic Joint/LConn1 -- strut_F/RConn1
  Prismatic Joint/RConn1 -- strut_M/RConn1
  Prismatic Joint/RConn2 -- PS-Simulink Converter/LConn1
  Simulink-PS Converter/RConn1 -- Prismatic Joint/LConn2
  Prismatic Joint/RConn3 -- PS-Simulink Converter1/LConn1

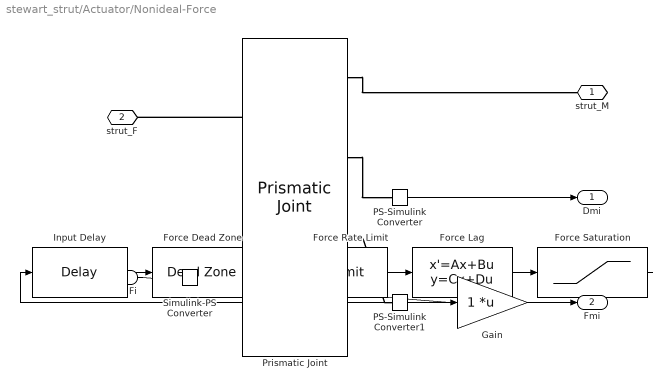
== system stewart_strut/Actuator/Nonideal-Force ==
  Fi : Inport
  Force Dead Zone : DeadZone  LowerValue=-stewart.nonidealForceActuator.deadzone(i)  UpperValue=stewart.nonidealForceActuator.deadzone(i)
  Force Lag : StateSpace  A=-1/stewart.nonidealForceActuator.timeConstant  B=1/stewart.nonidealForceActuator.timeConstant  D=0  InitialCondition=stewart.nonidealForceActuator.initialForce(i)
  Force Rate Limit : RateLimiter  RisingSlewLimit=stewart.nonidealForceActuator.forceRateLimit(i)  FallingSlewLimit=-stewart.nonidealForceActuator.forceRateLimit(i)  SampleTimeMode=inherited  InitialCondition=stewart.nonidealForceActuator.initialForce(i)
  Force Saturation : Saturate  UpperLimit=stewart.nonidealForceActuator.forceLimit(i)  LowerLimit=-stewart.nonidealForceActuator.forceLimit(i)
  Gain : Gain  Multiplication=Matrix(K*u)
  Input Delay : TransportDelay  DelayTime=stewart.nonidealForceActuator.inputDelay  InitialOutput=stewart.nonidealForceActuator.initialForce(i)
  PS-Simulink Converter : nesl_utility/PS-Simulink Converter  PhysicalDomain=network_engine_domain  SubClassName=ps_output  LeftPortType=input  RightPortType=output  PseudoPeriodic=off  Frequencies=[]  VectorFormat=1-D array  Unit=m  AffineConversion=off
  PS-Simulink Converter1 : nesl_utility/PS-Simulink Converter  PhysicalDomain=network_engine_domain  SubClassName=ps_output  LeftPortType=input  RightPortType=output  PseudoPeriodic=off  Frequencies=[]  VectorFormat=1-D array  Unit=N  AffineConversion=on
  Prismatic Joint : sm_lib/Joints/Prismatic Joint  JointMode=Normal  CompositeWrenchDir=BaseOnFollower  CompositeWrenchFrame=BaseFrame  SenseConstraintForce=off  SenseConstraintTorque=off  SenseTotalForce=on  SenseTotalTorque=off  PositionTargetSpecify=on  PositionTargetPriority=High  PositionTargetValue=stewart.actuators.Leq(i)  PositionTargetValueUnits=m  VelocityTargetSpecify=off  VelocityTargetPriority=High  VelocityTargetValue=0  VelocityTargetValueUnits=m/s  EquilibriumPosition=stewart.actuators.Leq(i)  EquilibriumPositionUnits=m  SpringStiffness=stewart.actuators.K(i)  SpringStiffnessUnits=N/m  DampingCoefficient=stewart.actuators.C(i)  DampingCoefficientUnits=N/(m/s)  LowerLimitSpecify=off  LowerLimitBound=-1  LowerLimitBoundUnits=m  LowerLimitStiffness=1e6  LowerLimitStiffnessUnits=N/m  LowerLimitDamping=1e3  LowerLimitDampingUnits=N/(m/s)  LowerLimitTransitionRegionWidth=1e-4  LowerLimitTransitionRegionWidthUnits=m  UpperLimitSpecify=off  UpperLimitBound=1  UpperLimitBoundUnits=m  UpperLimitStiffness=1e6  UpperLimitStiffnessUnits=N/m  UpperLimitDamping=1e3  UpperLimitDampingUnits=N/(m/s)  UpperLimitTransitionRegionWidth=1e-4  UpperLimitTransitionRegionWidthUnits=m  TorqueActuationMode=InputTorque  MotionActuationMode=ComputedMotion  SensePosition=on  SenseVelocity=off  SenseAcceleration=off  SenseTorqueForce=on  SenseLowerLimitTorqueForce=off  SenseUpperLimitTorqueForce=off
  Simulink-PS Converter : nesl_utility/Simulink-PS Converter  PhysicalDomain=network_engine_domain  SubClassName=ps_input  LeftPortType=input  RightPortType=output  PseudoPeriodic=off  Frequencies=[]  NoiseDistribution=none  NoiseParameters=[]  Unit=N  AffineConversion=off  FilteringAndDerivatives=provide  SimscapeFilterOrder=1  InputFilterTimeConstant=0.001  UdotUserProvided=0
  strut_M : PMIOPort  Side=Right
  strut_F : PMIOPort  Port=2  Side=Left
  Dmi : Outport
  Fmi : Outport  Port=2
  wires:
  PS-Simulink Converter/1 -> Dmi/1
  Fi/1 -> Gain/1
  Gain/1 -> Input Delay/1
  Input Delay/1 -> Force Dead Zone/1
  Force Dead Zone/1 -> Force Rate Limit/1
  Force Rate Limit/1 -> Force Lag/1
  Force Lag/1 -> Force Saturation/1
  Force Saturation/1 -> Simulink-PS Converter/1
  PS-Simulink Converter1/1 -> Fmi/1
  connections:
  Prismatic Joint/LConn1 -- strut_F/RConn1
  Prismatic Joint/LConn2 -- Simulink-PS Converter/RConn1
  Prismatic Joint/RConn1 -- strut_M/RConn1
  Prismatic Joint/RConn2 -- PS-Simulink Converter/LConn1
  Prismatic Joint/RConn3 -- PS-Simulink Converter1/LConn1

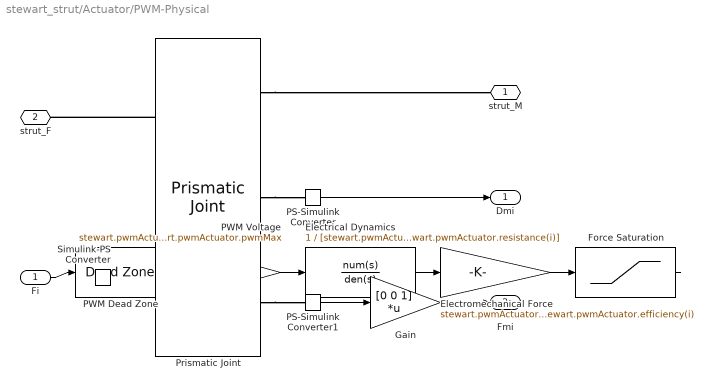
== system stewart_strut/Actuator/PWM-Physical ==
  Fi : Inport
  Electrical Dynamics : TransferFcn  Numerator=1  Denominator=[stewart.pwmActuator.inductance(i), stewart.pwmActuator.resistance(i)]
  Electromechanical Force : Gain  Gain=stewart.pwmActuator.torqueConstant(i)*stewart.pwmActuator.gearRatio(i)*2*pi/stewart.pwmActuator.screwLead(i)*stewart.pwmActuator.efficiency(i)
  Force Saturation : Saturate  UpperLimit=stewart.pwmActuator.forceLimit(i)  LowerLimit=-stewart.pwmActuator.forceLimit(i)
  Gain : Gain  Gain=[0 0 1]  Multiplication=Matrix(K*u)
  PS-Simulink Converter : nesl_utility/PS-Simulink Converter  PhysicalDomain=network_engine_domain  SubClassName=ps_output  LeftPortType=input  RightPortType=output  PseudoPeriodic=off  Frequencies=[]  VectorFormat=1-D array  Unit=m  AffineConversion=off
  PS-Simulink Converter1 : nesl_utility/PS-Simulink Converter  PhysicalDomain=network_engine_domain  SubClassName=ps_output  LeftPortType=input  RightPortType=output  PseudoPeriodic=off  Frequencies=[]  VectorFormat=1-D array  Unit=N  AffineConversion=on
  PWM Dead Zone : DeadZone  LowerValue=-stewart.pwmActuator.deadzonePwm(i)  UpperValue=stewart.pwmActuator.deadzonePwm(i)
  PWM Voltage : Gain  Gain=stewart.pwmActuator.busVoltage(i)/stewart.pwmActuator.pwmMax
  Prismatic Joint : sm_lib/Joints/Prismatic Joint  JointMode=Normal  CompositeWrenchDir=BaseOnFollower  CompositeWrenchFrame=BaseFrame  SenseConstraintForce=off  SenseConstraintTorque=off  SenseTotalForce=on  SenseTotalTorque=off  PositionTargetSpecify=on  PositionTargetPriority=High  PositionTargetValue=stewart.actuators.Leq(i)  PositionTargetValueUnits=m  VelocityTargetSpecify=off  VelocityTargetPriority=High  VelocityTargetValue=0  VelocityTargetValueUnits=m/s  EquilibriumPosition=stewart.actuators.Leq(i)  EquilibriumPositionUnits=m  SpringStiffness=stewart.actuators.K(i)  SpringStiffnessUnits=N/m  DampingCoefficient=stewart.actuators.C(i)  DampingCoefficientUnits=N/(m/s)  LowerLimitSpecify=off  LowerLimitBound=-1  LowerLimitBoundUnits=m  LowerLimitStiffness=1e6  LowerLimitStiffnessUnits=N/m  LowerLimitDamping=1e3  LowerLimitDampingUnits=N/(m/s)  LowerLimitTransitionRegionWidth=1e-4  LowerLimitTransitionRegionWidthUnits=m  UpperLimitSpecify=off  UpperLimitBound=1  UpperLimitBoundUnits=m  UpperLimitStiffness=1e6  UpperLimitStiffnessUnits=N/m  UpperLimitDamping=1e3  UpperLimitDampingUnits=N/(m/s)  UpperLimitTransitionRegionWidth=1e-4  UpperLimitTransitionRegionWidthUnits=m  TorqueActuationMode=InputTorque  MotionActuationMode=ComputedMotion  SensePosition=on  SenseVelocity=off  SenseAcceleration=off  SenseTorqueForce=off  SenseLowerLimitTorqueForce=off  SenseUpperLimitTorqueForce=off
  Simulink-PS Converter : nesl_utility/Simulink-PS Converter  PhysicalDomain=network_engine_domain  SubClassName=ps_input  LeftPortType=input  RightPortType=output  PseudoPeriodic=off  Frequencies=[]  NoiseDistribution=none  NoiseParameters=[]  Unit=N  AffineConversion=off  FilteringAndDerivatives=provide  SimscapeFilterOrder=1  InputFilterTimeConstant=0.001  UdotUserProvided=0
  strut_M : PMIOPort  Side=Right
  strut_F : PMIOPort  Port=2  Side=Left
  Dmi : Outport
  Fmi : Outport  Port=2
  wires:
  PS-Simulink Converter/1 -> Dmi/1
  PS-Simulink Converter1/1 -> Gain/1
  Gain/1 -> Fmi/1
  Fi/1 -> PWM Dead Zone/1
  PWM Dead Zone/1 -> PWM Voltage/1
  PWM Voltage/1 -> Electrical Dynamics/1
  Electrical Dynamics/1 -> Electromechanical Force/1
  Electromechanical Force/1 -> Force Saturation/1
  Force Saturation/1 -> Simulink-PS Converter/1
  connections:
  Prismatic Joint/LConn1 -- strut_F/RConn1
  Prismatic Joint/LConn2 -- Simulink-PS Converter/RConn1
  Prismatic Joint/RConn1 -- strut_M/RConn1
  Prismatic Joint/RConn2 -- PS-Simulink Converter/LConn1
  Prismatic Joint/RConn3 -- PS-Simulink Converter1/LConn1

== system stewart_strut/Inertial_Sensor/Accelerometer ==
  Brick Solid : sm_lib/Body Elements/Brick Solid  BrickDimensions=[1 1 1]  BrickDimensionsUnits=mm  ExportEntireGeometry=off  InertiaType=PointMass  BasedOnType=Density  Density=1000  DensityUnits=kg/m^3  Mass=stewart.sensors.inertial.M  MassUnits=kg  CenterOfMass=[0 0 0]  CenterOfMassUnits=m  MomentsOfInertia=[1 1 1]  MomentsOfInertiaUnits=kg*m^2  ProductsOfInertia=[0 0 0]  ProductsOfInertiaUnits=kg*m^2  GraphicType=FromGeometry  MarkerShape=Sphere  MarkerSize=10  GraphicVisPropType=SimpleVisualProperties  GraphicDiffuseColor=[0.5 0.5 0.5]  GraphicOpacity=1.0  GraphicSpecularColor=[0.5 0.5 0.5 1.0]  GraphicAmbientColor=[0.15 0.15 0.15 1.0]  GraphicEmissiveColor=[0.0 0.0 0.0 1.0]  GraphicShininess=75  DoExposeReferenceFrame=on  SerializedFrames=<Frames/>
  Gain : Gain  Gain=stewart.sensors.inertial.G
  Integrator : Integrator
  PS-Simulink Converter2 : nesl_utility/PS-Simulink Converter  PhysicalDomain=network_engine_domain  SubClassName=ps_output  LeftPortType=input  RightPortType=output  PseudoPeriodic=off  Frequencies=[]  VectorFormat=1-D array  Unit=m  AffineConversion=off
  Prismatic Joint : sm_lib/Joints/Prismatic Joint  JointMode=Normal  CompositeWrenchDir=FollowerOnBase  CompositeWrenchFrame=BaseFrame  SenseConstraintForce=off  SenseConstraintTorque=off  SenseTotalForce=off  SenseTotalTorque=off  PositionTargetSpecify=off  PositionTargetPriority=High  PositionTargetValue=0  PositionTargetValueUnits=m  VelocityTargetSpecify=off  VelocityTargetPriority=High  VelocityTargetValue=0  VelocityTargetValueUnits=m/s  EquilibriumPosition=0  EquilibriumPositionUnits=m  SpringStiffness=stewart.sensors.inertial.K  SpringStiffnessUnits=N/m  DampingCoefficient=stewart.sensors.inertial.C  DampingCoefficientUnits=N/(m/s)  LowerLimitSpecify=off  LowerLimitBound=-1  LowerLimitBoundUnits=m  LowerLimitStiffness=1e6  LowerLimitStiffnessUnits=N/m  LowerLimitDamping=1e3  LowerLimitDampingUnits=N/(m/s)  LowerLimitTransitionRegionWidth=1e-4  LowerLimitTransitionRegionWidthUnits=m  UpperLimitSpecify=off  UpperLimitBound=1  UpperLimitBoundUnits=m  UpperLimitStiffness=1e6  UpperLimitStiffnessUnits=N/m  UpperLimitDamping=1e3  UpperLimitDampingUnits=N/(m/s)  UpperLimitTransitionRegionWidth=1e-4  UpperLimitTransitionRegionWidthUnits=m  TorqueActuationMode=NoTorque  MotionActuationMode=ComputedMotion  SensePosition=on  SenseVelocity=off  SenseAcceleration=off  SenseTorqueForce=off  SenseLowerLimitTorqueForce=off  SenseUpperLimitTorqueForce=off
  B : PMIOPort  Side=Left
  Vmi : Outport
  wires:
  Integrator/1 -> Vmi/1
  Gain/1 -> Integrator/1
  PS-Simulink Converter2/1 -> Gain/1
  connections:
  Prismatic Joint/LConn1 -- B/RConn1
  Prismatic Joint/RConn2 -- PS-Simulink Converter2/LConn1
  Prismatic Joint/RConn1 -- Brick Solid/RConn1

== system stewart_strut/Inertial_Sensor/Geophone ==
  Brick Solid : sm_lib/Body Elements/Brick Solid  BrickDimensions=[1 1 1]  BrickDimensionsUnits=mm  ExportEntireGeometry=off  InertiaType=PointMass  BasedOnType=Density  Density=1000  DensityUnits=kg/m^3  Mass=stewart.sensors.inertial.M  MassUnits=kg  CenterOfMass=[0 0 0]  CenterOfMassUnits=m  MomentsOfInertia=[1 1 1]  MomentsOfInertiaUnits=kg*m^2  ProductsOfInertia=[0 0 0]  ProductsOfInertiaUnits=kg*m^2  GraphicType=FromGeometry  MarkerShape=Sphere  MarkerSize=10  GraphicVisPropType=SimpleVisualProperties  GraphicDiffuseColor=[0.5 0.5 0.5]  GraphicOpacity=1.0  GraphicSpecularColor=[0.5 0.5 0.5 1.0]  GraphicAmbientColor=[0.15 0.15 0.15 1.0]  GraphicEmissiveColor=[0.0 0.0 0.0 1.0]  GraphicShininess=75  DoExposeReferenceFrame=on  SerializedFrames=<Frames/>
  PS-Simulink Converter2 : nesl_utility/PS-Simulink Converter  PhysicalDomain=network_engine_domain  SubClassName=ps_output  LeftPortType=input  RightPortType=output  PseudoPeriodic=off  Frequencies=[]  VectorFormat=1-D array  Unit=m/s  AffineConversion=off
  Prismatic Joint : sm_lib/Joints/Prismatic Joint  JointMode=Normal  CompositeWrenchDir=FollowerOnBase  CompositeWrenchFrame=BaseFrame  SenseConstraintForce=off  SenseConstraintTorque=off  SenseTotalForce=off  SenseTotalTorque=off  PositionTargetSpecify=off  PositionTargetPriority=High  PositionTargetValue=0  PositionTargetValueUnits=m  VelocityTargetSpecify=off  VelocityTargetPriority=High  VelocityTargetValue=0  VelocityTargetValueUnits=m/s  EquilibriumPosition=0  EquilibriumPositionUnits=m  SpringStiffness=stewart.sensors.inertial.K  SpringStiffnessUnits=N/m  DampingCoefficient=stewart.sensors.inertial.C  DampingCoefficientUnits=N/(m/s)  LowerLimitSpecify=off  LowerLimitBound=-1  LowerLimitBoundUnits=m  LowerLimitStiffness=1e6  LowerLimitStiffnessUnits=N/m  LowerLimitDamping=1e3  LowerLimitDampingUnits=N/(m/s)  LowerLimitTransitionRegionWidth=1e-4  LowerLimitTransitionRegionWidthUnits=m  UpperLimitSpecify=off  UpperLimitBound=1  UpperLimitBoundUnits=m  UpperLimitStiffness=1e6  UpperLimitStiffnessUnits=N/m  UpperLimitDamping=1e3  UpperLimitDampingUnits=N/(m/s)  UpperLimitTransitionRegionWidth=1e-4  UpperLimitTransitionRegionWidthUnits=m  TorqueActuationMode=NoTorque  MotionActuationMode=ComputedMotion  SensePosition=off  SenseVelocity=on  SenseAcceleration=off  SenseTorqueForce=off  SenseLowerLimitTorqueForce=off  SenseUpperLimitTorqueForce=off
  B : PMIOPort  Side=Left
  Vmi : Outport
  wires:
  PS-Simulink Converter2/1 -> Vmi/1
  connections:
  Prismatic Joint/LConn1 -- B/RConn1
  Prismatic Joint/RConn2 -- PS-Simulink Converter2/LConn1
  Prismatic Joint/RConn1 -- Brick Solid/RConn1

== system stewart_strut/Inertial_Sensor/None ==
  Constant : Constant  Value=0
  B : PMIOPort  Side=Left
  Vmi : Outport
  wires:
  Constant/1 -> Vmi/1

== system stewart_strut/Joint_F/Flexible_Joint ==
  Reduced Order Flexible Solid : sm_lib/Body Elements/Flexible Bodies/Reduced Order Flexible Solid  UnitSystemType=SI  LengthUnit=m  MassUnit=kg  TimeUnit=s  NumberOfInterfaceFrames=2  InterfaceFrameOrigins=zeros(2,3)  InterfaceFrameOrientations=repmat([1 0 0 0],2,1)  StiffnessMatrix=stewart.joints_F.K  MassMatrix=stewart.joints_F.M  DampingType=UniformModal  ProportionalDampingAlpha=0  ProportionalDampingBeta=0.001  UniformModalDampingRatio=stewart.joints_F.xi  DampingMatrix=[]  ReferenceConditionsType=LinearizedMeanAxes  DoExposeReferenceFrame=off  ReductionType=None  NumRetainedModes=1  GraphicType=PartitionedGeometry  GeomFileName=mat/flexor_025.step  GeomUnitType=FromFile  VisRecursionLimit=3  GraphicVertexCoordinates=[]  GraphicFacetVertexIndices=[]  GraphicReconstructionMatrix=[]  GraphicVisPropType=FromFileVisualProperties  GraphicDiffuseColor=[0.5 0.5 0.5]  GraphicOpacity=1.0  GraphicSpecularColor=[0.5 0.5 0.5 1.0]  GraphicAmbientColor=[0.15 0.15 0.15 1.0]  GraphicEmissiveColor=[0.0 0.0 0.0 1.0]  GraphicShininess=75
  Ai : PMIOPort  Side=Left
  joint_F : PMIOPort  Port=2  Side=Right
  connections:
  Reduced Order Flexible Solid/LConn1 -- joint_F/RConn1
  Reduced Order Flexible Solid/RConn1 -- Ai/RConn1

== system stewart_strut/Joint_F/None ==
  Ai : PMIOPort  Side=Left
  joint_F : PMIOPort  Port=2  Side=Right
  connections:
  Ai/RConn1 -- joint_F/RConn1
